simulink model "consigna_5_2"  (R2024b)
settings: Solver=ode45  StartTime=0.0  StopTime=600  FixedStep=1/39789  MaxStep=1e-1  RelTol=1e-5
InitFcn:
  | parametros
values from neighbouring files (symbols this model uses):
  A_corrientes = [0 1; -omega_n_corrientes^2 -2*omega_n_corrientes]    [parametros.m]
  A_inversor = [0 1; -omega_n_inversor^2 -2*omega_n_inversor]    [parametros.m]
  A_posicion = [0 1; -omega_n_posicion^2 -2*omega_n_posicion]    [parametros.m]
  A_temp = -1/20    (= -0.05)    [parametros.m]
  alpha_cu = 3.9 *10^-3    (= 0.0039)    [parametros.m]
  B_corrientes = [0; omega_n_corrientes^2]    [parametros.m]
  B_inversor = [0; omega_n_inversor^2]    [parametros.m]
  b_l = 0.1    [parametros.m]
  b_m = 1.5 * 10^-5    (= 1.5e-05)    [parametros.m]
  B_posicion = [0; omega_n_posicion^2]    [parametros.m]
  B_temp = 1/20    (= 0.05)    [parametros.m]
  ba = J_eq*n*omega_pos    (= 0.0395694444444)    [parametros.m]
  C_corrientes = [1 0]    [parametros.m]
  C_inversor = [1 0]    [parametros.m]
  C_posicion = [1 0]    [parametros.m]
  C_temp = 1    [parametros.m]
  C_ts = 0.818    [parametros.m]
  J_l = (m*l_cm^2 + J_cm) + (m_l * l_l^2)    (= 0.0833)    [parametros.m]
  J_m = 1.4 * 10^-5    (= 1.4e-05)    [parametros.m]
  K_e_int = 3200 ^3    (= 32768000000)    [parametros.m]
  K_e_omega = 3*3200^2    (= 30720000)    [parametros.m]
  K_e_theta = 9600    [parametros.m]
  k_l = m * g * l_cm + m_l * g * l_l    (= 2.4516625)    [parametros.m]
  Ksa = J_eq*n*(omega_pos^2)    (= 31.6555555556)    [parametros.m]
  Ksia = J_eq*(omega_pos^3)    (= 10129.7777778)    [parametros.m]
  L_d = 6.6 * 10^-3    (= 0.0066)    [parametros.m]
  L_ls = 0.8 * 10^-3    (= 0.0008)    [parametros.m]
  L_q = 5.8 * 10^-3    (= 0.0058)    [parametros.m]
  lambda_m = 0.016    [parametros.m]
  P_p = 3    [parametros.m]
  r = 120    [parametros.m]
  R_s_40 = 1.02    [parametros.m]
  R_ts_amb = 146.7    [parametros.m]
  T_sample = 1/f_sample    (= 4.53514739229e-05)    [parametros.m]
  Temp_s_ref = 20    [parametros.m]
  tm = X(1)    [parametros.m]
  tr = X(2)    [parametros.m]
  w1 = 2*pi*r/5    (= 150.796447372)    [parametros.m]
  x0_corrientes = [0;0]    [parametros.m]
  x0_inversor = [0;0]    [parametros.m]
  x0_posicion = [0; 0]    [parametros.m]
  x0_temp = 25    [parametros.m]
libraries: simulink x23, dspsigops x6
(part 1 of 5)
settings Model: SimulationMode=accelerator  Creator=Usuario  LastModifiedBy=gabri
settings DebuggingCC: AlgebraicLoopMsg=none

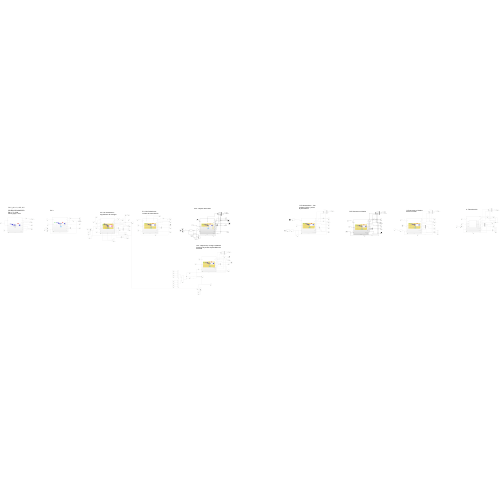
[thumbnail: Simulink's stored preview of the top-level diagram]
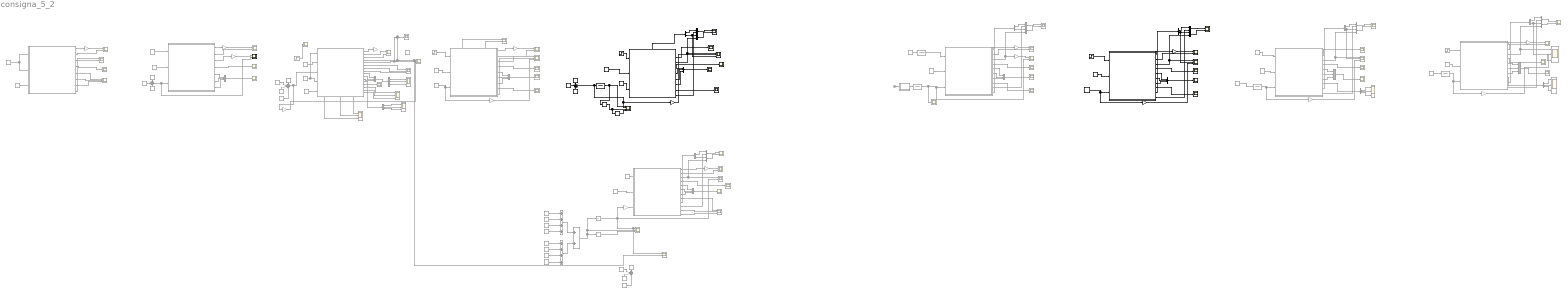
== system consigna_5_2 ==
  note: 5.2.1 i_ds* = 0, +0.5, -0.5
      |
      | PRUEBA SEGUIMIENTO TM* -> TL CON THETA_M(0) = PI/4
  note: 5.2.4 sin limitaciones - seguimiento de consigna
  note: 5.2.4 sin limitaciones - rechazo de perturbación
  note: 5.2.5 - Mejoras de consigna mediante formación de perfiles trapezoidales de velocidad
  note: 5.2.5 calentamiento - 10m consigna ciclica + pulsos de perturbación
  note: 5.2.5 Sensores no ideales
  note: 5.2.5 sensores no ideales inversor no ideal
  note: 6 - Discretización
  note: 5.2.3
  note: 5.2.5 - Mejora observador
  .5s : Step  Commented=on  Time=.5  After=5  SampleTime=0
  0-1 : simulink/Sources/Ramp  Commented=on  slope=2*pi/5  start=0  InitialOutput=0
  0-2 : simulink/Sources/Ramp  slope=2*pi/5  start=0  InitialOutput=0
  0-3 : simulink/Sources/Ramp  Commented=on  slope=2*pi/5  start=15  InitialOutput=0
  0-4 : simulink/Sources/Ramp  Commented=on  slope=2*pi/5  start=0  InitialOutput=0
  0-5 : simulink/Sources/Ramp  Commented=on  slope=2*pi/5  start=0  InitialOutput=0
  0-6 : simulink/Sources/Ramp  Commented=on  slope=2*pi/5  start=15  InitialOutput=0
  10-1 : simulink/Sources/Ramp  Commented=on  slope=-2*pi/5  start=10  InitialOutput=0
  10-15 : simulink/Sources/Ramp  Commented=on  slope=-2*pi/5  start=10  InitialOutput=0
  10-2 : simulink/Sources/Ramp  slope=-2*pi/5  start=10  InitialOutput=0
  10-3 : simulink/Sources/Ramp  Commented=on  slope=-2*pi/5  start=10  InitialOutput=0
  5-1 : simulink/Sources/Ramp  Commented=on  slope=-2*pi/5  start=5  InitialOutput=0
  5-10 : simulink/Sources/Ramp  Commented=on  slope=-2*pi/5  start=5  InitialOutput=0
  5-2 : simulink/Sources/Ramp  slope=-2*pi/5  start=5  InitialOutput=0
  5-3 : simulink/Sources/Ramp  Commented=on  slope=-2*pi/5  start=5  InitialOutput=0
  "5.2.1 " : Subsystem  Commented=on
  5.2.3 : Subsystem  Commented=on
  5.2.4 : Subsystem  Commented=on
      settings: PortSchema="{\"entries\":[{\"content\":{\"sides\":[{\"content\":{\"connectorIds\":[\"In1\",\"In2\",\"In3\",\"In4\",\"In5\"]},\"type\":\"ConnectorPlacement.EquallySpacedRectSide\",\"uuid\":\"f25aa34c-6f67-484c-a229-f52c6eeecdf1\"},{\"content\":{\"connectorIds\":[\"Out1\",\"Out2\",\"Out3\",\"Out4\",\"Out5\",\"Out6\",\"Out7\",\"Out8\",\"Out9\",\"Out10\",\"Out11\",\"Out12\",\"Out13\",\"Out14\",\"Out15\",\"Out16\"],\"side\":\"RIGHT\"},\"type\":\"ConnectorPlacement.EquallySpacedRectSide\",\"uuid\":\"6aed1817-4278-445a-93c2-caff5363bf6f\"},{\"content\":{\"side\":\"TOP\"},\"type\":\"ConnectorPlacement.EquallySpacedRectSide\",\"uuid\":\"7cbfa292-0843-4ea0-b7b1-1b35692a06de\"},{\"content\":{\"connectorIds\":[\"Out17\",\"Out18\",\"Out19\"],\"side\":\"BOTTOM\"},\"type\":\"ConnectorPlacement.EquallySpacedRectSide\",\"uuid\":\"b199e458-5f17-4edf-b279-750495dc0f0e\"}]},\"type\":\"ConnectorPlacement.EquallySpacedConnector\",\"uuid\":\"19aabd2c-ee83-4195-b5ac-13c3d5f141f0\"}],\"packageUris\":[\"http://schema.mathworks.com/mf0/Connector/R2020b\"],\"version\":\"1.0\"}"
  5.2.4.b : Subsystem  Commented=on
      settings: PortSchema="{\"entries\":[{\"content\":{\"sides\":[{\"content\":{\"connectorIds\":[\"In1\",\"In2\",\"In3\"]},\"type\":\"ConnectorPlacement.EquallySpacedRectSide\",\"uuid\":\"8b25de47-475f-4287-8ae4-53eaf326d459\"},{\"content\":{\"connectorIds\":[\"Out1\",\"Out2\",\"Out3\",\"Out4\",\"Out5\",\"Out6\",\"Out7\",\"Out8\",\"Out9\"],\"side\":\"RIGHT\"},\"type\":\"ConnectorPlacement.EquallySpacedRectSide\",\"uuid\":\"f06d5897-8e36-455d-9b67-4a95e7a5221c\"},{\"content\":{\"connectorIds\":[\"Out10\",\"Out11\"],\"side\":\"TOP\"},\"type\":\"ConnectorPlacement.EquallySpacedRectSide\",\"uuid\":\"fe71d55b-b6d0-46da-a788-438a4a7d80b0\"}]},\"type\":\"ConnectorPlacement.EquallySpacedConnector\",\"uuid\":\"95d0947e-b21b-4577-be3e-7cfd2e0895b9\"}],\"packageUris\":[\"http://schema.mathworks.com/mf0/Connector/R2020b\"],\"version\":\"1.0\"}"
  5.2.5 : Subsystem
      settings: PortSchema="{\"entries\":[{\"content\":{\"sides\":[{\"content\":{\"connectorIds\":[\"In1\",\"In2\",\"In3\"]},\"type\":\"ConnectorPlacement.EquallySpacedRectSide\",\"uuid\":\"8b25de47-475f-4287-8ae4-53eaf326d459\"},{\"content\":{\"connectorIds\":[\"Out1\",\"Out2\",\"Out3\",\"Out4\",\"Out5\",\"Out6\",\"Out7\",\"Out8\",\"Out9\"],\"side\":\"RIGHT\"},\"type\":\"ConnectorPlacement.EquallySpacedRectSide\",\"uuid\":\"f06d5897-8e36-455d-9b67-4a95e7a5221c\"},{\"content\":{\"connectorIds\":[\"Out10\"],\"side\":\"TOP\"},\"type\":\"ConnectorPlacement.EquallySpacedRectSide\",\"uuid\":\"fe71d55b-b6d0-46da-a788-438a4a7d80b0\"}]},\"type\":\"ConnectorPlacement.EquallySpacedConnector\",\"uuid\":\"95d0947e-b21b-4577-be3e-7cfd2e0895b9\"}],\"packageUris\":[\"http://schema.mathworks.com/mf0/Connector/R2020b\"],\"version\":\"1.0\"}"
  5.2.5' : Subsystem  Commented=on
  5.2.5.c : Subsystem  Commented=on
  5.2.5.d : Subsystem
  5.2.5.e : Subsystem  Commented=on
  Clock : Clock  Commented=on
  Constant{,1,6,10..11} (5 alike) : Constant  Commented=on  Value=20
  Constant12 : Constant  Commented=on  Value=40
  Constant13 : Constant  Value=20
  Constant14 : Constant  Commented=on  Value=40
  Constant{3..4,15,17..22} (9 alike) : Constant  Commented=on  Value=0
  Constant16 : Constant  Value=0
  Constant2 : Constant  Commented=on  Value=40
  Constant5 : Constant  Value=20
  Constant9 : Constant  Value=0
  Demux : Demux  Outputs=2
  Demux{6..8,10} (4 alike) : Demux  Commented=on  Outputs=3
  Demux{2..3,5,9} (4 alike) : Demux  Commented=on  Outputs=2
  Demux4 : Demux  Outputs=2
  Derivative : Derivative
  Derivative1 : Derivative
  Derivative2 : Derivative  Commented=on
  Error de observador : Scope  NumInputPorts=2
  Error de observador{2..3,5..6} (4 alike) : Scope  Commented=on  NumInputPorts=2
  Error de observador4 : Scope  NumInputPorts=2
  Gain{,4..6,8,14..15,20..21,36} (10 alike) : Gain  Commented=on  Gain=1/r
  Gain{1,28,30,32} (4 alike) : Gain  Commented=on  Gain=r
  Gain2 : Gain  Gain=r
  Gain3 : Gain  Gain=r
  Gain7 : Gain  Gain=1/r
  Integrator : Integrator  Commented=on
  MATLAB Function : MATLAB Function  Commented=on  TreatAsAtomicUnit=on
  Mux{,4,14,16} (4 alike) : Mux  Inputs=2
  Mux{1..2,9,12,18,21,41} (7 alike) : Mux  Commented=on  Inputs=3
  Mux{8,10..11,13,17,19..20,22} (8 alike) : Mux  Commented=on  Inputs=2
  Mux15 : Mux  Inputs=3
  Mux3 : Mux  Inputs=3
  Posición y velocidad : Scope  Commented=on  NumInputPorts=2
  Pulse Generator : DiscretePulseGenerator  Commented=on  PulseType=Time based  Amplitude=5  Period=1  PulseWidth=50
  Ramp : simulink/Sources/Ramp  Commented=on  slope=3*pi  start=5  InitialOutput=0
  Ramp1 : simulink/Sources/Ramp  Commented=on  slope=-w1  start=15  InitialOutput=0
  Ramp2 : simulink/Sources/Ramp  Commented=on  slope=w1  start=10+tr+tm  InitialOutput=0
  Ramp3 : simulink/Sources/Ramp  Commented=on  slope=w1  start=10+tr  InitialOutput=0
  Ramp4 : simulink/Sources/Ramp  Commented=on  slope=-w1  start=10  InitialOutput=0
  Ramp5 : simulink/Sources/Ramp  Commented=on  slope=w1  start=5  InitialOutput=0
  Ramp6 : simulink/Sources/Ramp  Commented=on  slope=-w1  start=tr+tm  InitialOutput=0
  Ramp7 : simulink/Sources/Ramp  Commented=on  slope=-w1  start=tr  InitialOutput=0
  Ramp8 : simulink/Sources/Ramp  Commented=on  slope=w1  start=0  InitialOutput=0
  Scope : Scope  Commented=on  NumInputPorts=2
  Scope1 : Scope  NumInputPorts=4
  Scope11 : Scope  Commented=on
  Scope4 : Scope  Commented=on  NumInputPorts=3
  Step : Step  Time=7.5  After=5  SampleTime=0
  Step1 : Step  Commented=on  Time=7.5  After=5  SampleTime=0
  Step3 : Step  Commented=on  Time=7.5  After=5  SampleTime=0
  Step4 : Step  Time=7.5  After=5  SampleTime=0
  Subsystem : Subsystem  Commented=on
  Sum : Sum  Commented=on  Inputs=+++
  Sum{1,3,8,11} (4 alike) : Sum  Commented=on  Inputs=++++
  Sum2 : Sum  Commented=on  Inputs=|-+
  Sum6 : Sum  Inputs=+++
  Sum9 : Sum  Commented=on
  Temperatura : Scope  Commented=on
  Tensiones Virtuales : Scope  Commented=on  NumInputPorts=3
  Tensiones reales : Scope  Commented=on  NumInputPorts=3
  Tensiones1 : Scope  Commented=on
  Tensiones2 : Scope
  Tensiones4 : Scope  Commented=on  NumInputPorts=3
  Tensiones5 : Scope  Commented=on
  Tensiones6 : Scope
  Tensiones7 : Scope  Commented=on  NumInputPorts=3
  Tensiones8 : Scope  Commented=on  NumInputPorts=3
  Torque carga vs motor : Scope  Commented=on  NumInputPorts=2
  Transfer Fcn2 : TransferFcn  Numerator=[10]  Denominator=[1 10]
  Transfer Fcn3 : TransferFcn  Commented=on  Numerator=[100]  Denominator=[1 100]
  Transfer Fcn4 : TransferFcn  Commented=on  Numerator=[10]  Denominator=[1 10]
  Transfer Fcn5 : TransferFcn  Commented=on  Numerator=[10]  Denominator=[1 10]
  Transfer Fcn8 : TransferFcn  Commented=on  Numerator=[20]  Denominator=[1 20]
  corrientes : Scope  Commented=on  NumInputPorts=3
  corrientes virtuales : Scope  Commented=on  NumInputPorts=3
  corrientes{2..3,6..7,9..10} (6 alike) : Scope  Commented=on
  corrientes4 : Scope
  corrientes8 : Scope
  corrrientes reales : Scope  Commented=on  NumInputPorts=3
  error de posicion : Scope  Commented=on
  posicion : Scope  Commented=on  NumInputPorts=3
  posicion del brazo : Scope  NumInputPorts=2
  posicion del brazo5 : Scope  Commented=on  NumInputPorts=2
  posicion del brazo6 : Scope  Commented=on  NumInputPorts=2
  posicion del brazo7 : Scope  NumInputPorts=3
  posicion del brazo8 : Scope  Commented=on  NumInputPorts=3
  posicion del brazo9 : Scope  Commented=on  NumInputPorts=3
  posicion2 : Scope  NumInputPorts=3
  posicion3 : Scope  Commented=on  NumInputPorts=3
  temp{,1..2,5..6,8..9} (7 alike) : Scope  Commented=on
  temp3 : Scope
  temp7 : Scope
  tld : Scope  Commented=on
  torque{,1..2,5..6,9} (6 alike) : Scope  Commented=on  NumInputPorts=2
  torque3 : Scope
  torque7 : Scope  NumInputPorts=2
  torque8 : Scope  Commented=on
  "velocidad " : Scope  Commented=on  NumInputPorts=2
  velocidad del brazo : Scope  Commented=on  NumInputPorts=3
  wires:
  5.2.3/7(fcs) -> Mux41/3
  5.2.3/5(fas) -> Mux41/1
  5.2.3/6(fbs) -> Mux41/2
  Mux41/1 -> corrientes2/1
  5.2.3/3("theta_m ") -> Gain/1
  Constant/1 -> 5.2.3/2(Tº_amb)
  5.2.3/4(T_s) -> temp/1
  "5.2.1 "/3("theta_m ") -> Posición y velocidad/1  "theta_m"
  Constant6/1 -> "5.2.1 "/3(Tº_amb)
  "5.2.1 "/7(fcs) -> corrientes/3  "i_cs"
  "5.2.1 "/6(fbs) -> corrientes/2  "i_bs"
  "5.2.1 "/2(T_m) -> Torque carga vs motor/2  "T_m"
  "5.2.1 "/5(fas) -> corrientes/1  "i_as"
  "5.2.1 "/4(T_s) -> Temperatura/1  "T_s"
  5.2.3/2(T_m) -> torque/2
  Sum/1 -> posicion del brazo/2, 5.2.3/3(q1*)  "q1*"
  0-5/1 -> Sum/2
  Gain/1 -> posicion del brazo/1  "q1"
  5-10/1 -> Sum/1
  10-15/1 -> Sum/3
  5-1/1 -> Sum1/1
  0-1/1 -> Sum1/2
  5.2.4/2(T_m) -> torque1/1  "Tm"
  5.2.4/4("theta_m ") -> Sum2/2, Scope/2, posicion/1  "theta_m"
  10-1/1 -> Sum1/3
  Mux1/1 -> Demux7/1
  5.2.4/13(T_s) -> temp1/1
  5.2.4/11(fcs) -> Mux1/3
  5.2.4/10(fbs) -> Mux1/2
  Constant1/1 -> 5.2.4/2(Tº_amb)
  5.2.4/9(fas) -> Mux1/1
  5.2.4/12(v_abcs) -> Demux6/1
  "5.2.1 "/8(omega_m) -> Posición y velocidad/2  "omega_m"
  5.2.4.b/5(fas) -> Mux2/1
  Step1/1 -> 5.2.4.b/1(T_per)  "T_per"
  Constant2/1 -> 5.2.4.b/2(Tº_amb)
  5.2.4.b/4(T_s) -> temp2/1
  5.2.4.b/2(T_m) -> torque2/2  "Tm"
  5.2.4.b/7(fcs) -> Mux2/3
  5.2.4.b/6(fbs) -> Mux2/2
  5.2.4.b/8(v_abcs) -> Tensiones1/1
  Mux2/1 -> corrientes3/1
  Constant3/1 -> Gain1/1, 5.2.4.b/3(q1*)  "q1*"
  Step3/1 -> tld/1
  Mux3/1 -> corrientes4/1  "i_abcs"
  5.2.5/7(fcs) -> Mux3/3  "ics"
  Sum6/1 -> Transfer Fcn2/1, Scope1/2, Gain2/1  "q1*"
  5.2.5/8(v_abcs) -> Tensiones2/1  "v_abcs"
  Constant5/1 -> 5.2.5/2(Tº_amb)
  5.2.5/5(fas) -> Mux3/1  "ias"
  5.2.5/6(fbs) -> Mux3/2  "ibs"
  5.2.5/2(T_m) -> torque3/1  "Tm"
  5.2.5/3("theta_m ") -> posicion2/1, Mux4/2  "theta_m"
  5.2.5/4(T_s) -> temp3/1  "T_s"
  Mux/1 -> Error de observador/1
  5.2.5/10(omega_theta_m_obs) -> Demux/1
  Demux/1 -> Mux/1  "omega_m_obs"
  5.2.5/9(omega_m) -> Mux/2  "omega_m"
  Demux/2 -> posicion2/3, Mux4/1  "theta_m_obs"
  Mux4/1 -> Error de observador/2
  5-2/1 -> Sum6/1
  0-2/1 -> Sum6/2
  10-2/1 -> Sum6/3
  Derivative/1 -> Derivative1/1, Scope1/3  "v"
  Derivative1/1 -> Scope1/4  "a"
  Constant9/1 -> 5.2.5/3(q1*)
  Transfer Fcn2/1 -> Scope1/1, Derivative/1  "q1* - suavizada"
  Transfer Fcn8/1 -> Scope11/1, posicion del brazo6/2, 5.2.5.c/3(q1*)  "q1*"
  Demux3/1 -> Mux13/1  "omega_m_obs"
  5.2.5.c/9(omega_m) -> Mux13/2  "omega_m"
  5.2.5.c/4(T_s) -> temp6/1  "T_s"
  5.2.5.c/10(omega_theta_obs) -> Demux3/1
  5.2.5.c/7(fcs) -> Mux12/3
  Mux12/1 -> corrientes7/1
  5.2.5.c/5(fas) -> Mux12/1
  5.2.5.c/8(v_abcs) -> Tensiones5/1
  Transfer Fcn3/1 -> 5.2.5.c/1(T_per)  "T_per"
  5.2.5.c/3("theta_m ") -> Mux11/2, Gain21/1  "theta_m"
  Demux3/2 -> Mux11/1  "theta_m_obs"
  Mux11/1 -> Error de observador3/2
  5.2.5.c/6(fbs) -> Mux12/2
  Mux13/1 -> Error de observador3/1
  5.2.5.c/2(T_m) -> torque6/2  "Tm"
  Gain21/1 -> posicion del brazo6/1  "q1"
  Constant11/1 -> 5.2.5.c/2(Tº_amb)
  Pulse Generator/1 -> Transfer Fcn3/1  "Tper"
  Demux4/2 -> posicion del brazo7/2, Mux14/1  "theta_m_obs"
  Constant13/1 -> 5.2.5.d/2(Tº_amb)
  5.2.5.d/3("theta_m ") -> Mux14/2, posicion del brazo7/1  "theta_m"
  5.2.5.d/2(T_m) -> torque7/2  "Tm"
  5.2.5.d/9(omega_theta_obs) -> Demux4/1
  5.2.5.d/4(T_s) -> temp7/1  "T_s"
  5.2.5.d/5(fas) -> Mux15/1  "i_as"
  5.2.5.d/6(fbs) -> Mux15/2  "i_bs"
  5.2.5.d/8(v_abcs) -> Tensiones6/1
  Step/1 -> 5.2.5.d/1(T_per)  "T_per"
  Mux14/1 -> Error de observador4/2
  Mux16/1 -> Error de observador4/1
  Mux15/1 -> corrientes8/1
  5.2.5.d/7(fcs) -> Mux15/3  "i_cs"
  5.2.5.d/10(omega_m) -> Mux16/2  "omega_m"
  5.2.4/6(omega_m_obs) -> velocidad del brazo/1  "omega_m_obs"
  5.2.4/7(omega_m) -> velocidad del brazo/2  "omega_m simulada"
  5.2.4/8(omega_m*) -> velocidad del brazo/3  "omega_m*"
  Demux6/1 -> Tensiones reales/1  "v_as"
  Demux6/2 -> Tensiones reales/2  "v_bs"
  Demux6/3 -> Tensiones reales/3  "v_cs"
  Demux7/1 -> corrrientes reales/1  "i_as"
  Demux7/2 -> corrrientes reales/2  "i_bs"
  Demux7/3 -> corrrientes reales/3  "i_cs"
  Clock/1 -> MATLAB Function/1(t)
  MATLAB Function/1(y) -> Transfer Fcn8/1
  Constant16/1 -> Gain3/1, 5.2.5.d/3(q1*)  "q1*"
  Gain3/1 -> posicion del brazo7/3  "theta_m*"
  Transfer Fcn4/1 -> Gain28/1, 5.2.5.e/3(q1*)  "q1*"
  Gain28/1 -> posicion del brazo8/3  "theta_m*"
  Mux19/1 -> Error de observador5/1
  5.2.5.e/8(v_abcs) -> Demux8/1
  5.2.5.e/5(fas) -> Mux18/1  "i_as"
  5.2.5.e/6(fbs) -> Mux18/2  "i_bs"
  Demux5/2 -> posicion del brazo8/2, Mux17/1  "theta_m_obs"
  Demux5/1 -> Mux19/1  "omega_m_obs"
  Mux17/1 -> Error de observador5/2
  5.2.5.e/10(omega_m) -> Mux19/2  "omega_m"
  Mux18/1 -> corrientes9/1
  5.2.5.e/3("theta_m ") -> Mux17/2, posicion del brazo8/1  "theta_m"
  5.2.5.e/7(fcs) -> Mux18/3  "i_cs"
  Constant15/1 -> 5.2.5.e/1(T_per)  "T_per"
  Constant12/1 -> 5.2.5.e/2(Tº_amb)
  5.2.5.e/2(T_m) -> torque8/1  "Tm"
  5.2.5.e/9(omega_theta_obs) -> Demux5/1
  5.2.5.e/4(T_s) -> temp8/1  "T_s"
  Ramp/1 -> Transfer Fcn4/1  "q1*"
  Demux8/1 -> Tensiones7/1  "v_as"
  Demux8/2 -> Tensiones7/2  "v_bs"
  Demux8/3 -> Tensiones7/3  "v_cs"
  Demux9/1 -> Mux22/1  "omega_m_obs"
  Mux20/1 -> Error de observador6/2
  Mux22/1 -> Error de observador6/1
  Mux21/1 -> corrientes10/1
  Demux9/2 -> posicion del brazo9/3, Mux20/1  "theta_m_obs"
  Gain32/1 -> posicion del brazo9/2  "theta_m*"
  Demux10/2 -> Tensiones8/2  "v_bs"
  Demux10/1 -> Tensiones8/1  "v_as"
  Constant20/1 -> Transfer Fcn5/1  "q1*"
  Demux10/3 -> Tensiones8/3  "v_cs"
  Transfer Fcn5/1 -> Subsystem/3(q1*), Gain32/1
  5.2.5'/4(T_s) -> temp5/1
  5.2.5'/9(omega_theta_obs) -> Demux2/1
  5.2.5'/2(T_m) -> torque5/2  "Tm"
  Mux9/1 -> corrientes6/1
  5.2.5'/7(fcs) -> Mux9/3  "ics"
  5.2.5'/10(omega_m) -> Mux8/2  "omega_m"
  5.2.5'/3("theta_m ") -> posicion del brazo5/1, Mux10/2  "theta_m"
  Constant18/1 -> 5.2.5'/1(T_per)
  Demux2/2 -> Mux10/1  "theta_m_obs"
  Mux10/1 -> Error de observador2/2
  Demux2/1 -> Mux8/1  "omega_m_obs"
  5.2.5'/6(fbs) -> Mux9/2  "ibs"
  5.2.5'/8(v_as) -> Tensiones4/1  "vas"
  Constant10/1 -> 5.2.5'/2(Tº_amb)
  5.2.5'/5(fas) -> Mux9/1  "ias"
  Mux8/1 -> Error de observador2/1
  Ramp1/1 -> Sum8/1
  Ramp4/1 -> Sum8/4
  Ramp3/1 -> Sum8/3
  Ramp2/1 -> Sum8/2
  Ramp8/1 -> Sum11/4
  Ramp7/1 -> Sum11/3
  Ramp6/1 -> Sum11/2
  Ramp5/1 -> Sum11/1
  Sum8/1 -> Sum9/1
  Sum11/1 -> Sum9/2
  Sum9/1 -> Derivative2/1, Integrator/1, Scope4/2  "vel"
  Integrator/1 -> posicion del brazo5/2, Gain36/1, Scope/1, Scope4/1  "Consigna de Posicion"
  Derivative2/1 -> Scope4/3  "acel"
  Constant17/1 -> 5.2.3/1(T_per)
  "5.2.1 "/1(T_l) -> Gain4/1
  Constant19/1 -> "5.2.1 "/1(Tm*), "5.2.1 "/2(T_per)
  5.2.4.b/1(T_l) -> Gain15/1
  5.2.4.b/9(theta_m_obs) -> posicion3/2  "theta_m_obs"
  5.2.4.b/3("theta_m ") -> posicion3/1  "theta_m"
  Gain1/1 -> posicion3/3  "theta_m*"
  Gain2/1 -> posicion2/2  "theta_m*"
  5.2.5'/1(T_l) -> Gain20/1
  Gain4/1 -> Torque carga vs motor/1  "T_l"
  5.2.3/1(T_l) -> Gain5/1
  Gain5/1 -> torque/1
  5.2.4/1(T_l) -> Gain14/1
  Gain15/1 -> torque2/1
  5.2.4.b/10(omega_m_simulada) -> "velocidad "/1
  5.2.4.b/11(omega_m_obs) -> "velocidad "/2
  Gain20/1 -> torque5/1  "q1"
  Gain36/1 -> 5.2.5'/3(q1*)
  5.2.5.c/1(T_l) -> Gain6/1
  Gain6/1 -> torque6/1  "q1"
  Demux4/1 -> Mux16/1
  5.2.5.d/1(T_l) -> Gain7/1
  Gain7/1 -> torque7/1  "theta_m*"
  Gain8/1 -> torque9/1
  Subsystem/3(theta_m) -> Mux20/2, posicion del brazo9/1  "theta_m muestreada"
  .5s/1 -> Subsystem/1(T_per)  "T_per"
  Constant14/1 -> Subsystem/2(Tº_amb)
  Subsystem/1(omega_m) -> Gain8/1
  Subsystem/2(Tm) -> torque9/2
  Subsystem/4(T_s) -> temp9/1  "T_s"
  Subsystem/5(i_as) -> Mux21/1
  Subsystem/6(i_bs) -> Mux21/2
  Subsystem/7(i_cs) -> Mux21/3
  Subsystem/8(v_abcs) -> Demux10/1
  Subsystem/9(omega_theta_obs) -> Demux9/1
  Subsystem/10(omega_m1) -> Mux22/2
  0-3/1 -> Sum1/4
  5.2.4/3(Tm*) -> torque1/2
  5.2.4/14(v_qs*') -> Tensiones Virtuales/1
  5.2.4/15(v_ds*') -> Tensiones Virtuales/2
  5.2.4/16(v_0s*') -> Tensiones Virtuales/3
  Constant21/1 -> 5.2.4/1(T_per), 5.2.4/4(I_ds*)
  Constant22/1 -> 5.2.4/5(I_0s*)
  5.2.4/19(iqs) -> corrientes virtuales/1
  5.2.4/18(ids) -> corrientes virtuales/2
  5.2.4/17(i0s) -> corrientes virtuales/3
  5.2.4/5(theta_m_obs) -> Sum2/1, posicion/2  "theta_m_obs"
  Sum2/1 -> error de posicion/1
  Sum1/1 -> Gain30/1, 5.2.4/3(q1*)  "q1*"
  Gain30/1 -> posicion/3  "theta_m*"
  10-3/1 -> Sum3/3
  0-6/1 -> Sum3/4
  0-4/1 -> Sum3/2
  5-3/1 -> Sum3/1
  5.2.5'/11(v_bs) -> Tensiones4/2  "vbs"
  5.2.5'/12(v_cs) -> Tensiones4/3  "vcs"
  Step4/1 -> 5.2.5/1(T_per)  "Tper"

== system consigna_5_2/5.2.1  ==
  Tm* : Inport
  T_per : Inport  Port=2
  Tº_amb : Inport  Port=3
  Calculo rs : Subsystem
  Constant5 : Constant  Value=0
  Demux : Demux  Outputs=3
  Desacoplamientos físicos : Subsystem
  Desacoplamientos físicos de torque : Subsystem
  Gain5 : Gain  Gain=P_p
  Modulador de corriente : Subsystem
  Modulador de tensión : Subsystem
  Modulador de torque : Subsystem
  Sensores : Subsystem
  Subsistema físico no lineal : Subsystem
      settings: PortSchema="{\"entries\":[{\"content\":{\"sides\":[{\"content\":{\"connectorIds\":[\"In1\",\"In2\",\"In3\",\"In4\",\"In5\"]},\"type\":\"ConnectorPlacement.EquallySpacedRectSide\",\"uuid\":\"67117692-d9ee-40bf-88b2-d8f6a60dc3b5\"},{\"content\":{\"connectorIds\":[\"Out1\",\"Out2\",\"Out3\"],\"side\":\"RIGHT\"},\"type\":\"ConnectorPlacement.EquallySpacedRectSide\",\"uuid\":\"ca2dbe86-e86f-47c7-8eac-1e82e6a5dbc0\"},{\"content\":{\"connectorIds\":[\"Out4\",\"Out5\",\"Out6\"],\"side\":\"TOP\"},\"type\":\"ConnectorPlacement.EquallySpacedRectSide\",\"uuid\":\"fbd4a5c3-5162-48dd-8002-932f8e6631f6\"}]},\"type\":\"ConnectorPlacement.EquallySpacedConnector\",\"uuid\":\"e55c07f0-88b9-4508-920f-2bf50421126b\"}],\"packageUris\":[\"http://schema.mathworks.com/mf0/Connector/R2020b\"],\"version\":\"1.0\"}"
  TD_PARK : MATLAB Function  TreatAsAtomicUnit=on
  TI_PARK1 : MATLAB Function  TreatAsAtomicUnit=on
  T_l : Outport
  T_m : Outport  Port=2
  "theta_m " : Outport  Port=3
  T_s : Outport  Port=4
  fas : Outport  Port=5
  fbs : Outport  Port=6
  fcs : Outport  Port=7
  omega_m : Outport  Port=8
  wires:
  Modulador de tensión/1(v_as) -> Subsistema físico no lineal/2(v_as)
  TD_PARK/3(f0s) -> Desacoplamientos físicos/6(i_0s), Modulador de corriente/6(i_0s)  "i_0s"
  TI_PARK1/1(fas) -> Modulador de tensión/1(v_as*)
  Sensores/2(T_s_medida) -> T_s/1, Calculo rs/1(Ts)
  Modulador de tensión/2(v_bs) -> Subsistema físico no lineal/3(v_bs)
  TD_PARK/1(fqs) -> Modulador de corriente/4(i_qs), Desacoplamientos físicos/4(i_qs)  "i_qs^r"
  Sensores/1(theta_m_medida) -> "theta_m "/1, Desacoplamientos físicos de torque/2(theta_m), Gain5/1
  TI_PARK1/2(fbs) -> Modulador de tensión/2(v_bs*)
  TD_PARK/2(fds) -> Modulador de torque/2(ids), Desacoplamientos físicos/5(i_ds), Modulador de corriente/5(i_ds)  "i_ds^r"
  Desacoplamientos físicos/3(v_0s*') -> TI_PARK1/3(f0s)
  Modulador de tensión/3(v_cs) -> Subsistema físico no lineal/4(v_cs)
  Subsistema físico no lineal/1(theta_m) -> Sensores/1(theta_m)
  Subsistema físico no lineal/2(T_s) -> Sensores/2(T_s)
  Sensores/5(i_cs_medida) -> fcs/1, TD_PARK/3(fcs)
  Demux/1 -> Sensores/3(i_as)
  Modulador de torque/1(iq*) -> Modulador de corriente/1(I_qs*)
  Gain5/1 -> TD_PARK/4(theta_r), TI_PARK1/4(theta_r)
  Sensores/4(i_bs_medida) -> fbs/1, TD_PARK/2(fbs)
  Modulador de corriente/1(v_qs*) -> Desacoplamientos físicos/1(v_qs*)
  Constant5/1 -> Modulador de corriente/3(I_0s*), Modulador de corriente/2(I_ds*)
  T_per/1 -> Subsistema físico no lineal/1(T_per)
  Demux/2 -> Sensores/4(i_bs)
  Modulador de corriente/3(v_0s*) -> Desacoplamientos físicos/3(v_0s*)
  Demux/3 -> Sensores/5(i_cs)
  Desacoplamientos físicos/1(v_qs*') -> TI_PARK1/1(fqs)
  Sensores/3(i_as_medida) -> TD_PARK/1(fas), fas/1
  TI_PARK1/3(fcs) -> Modulador de tensión/3(v_cs*)
  Tº_amb/1 -> Subsistema físico no lineal/5(Tº_amb), Calculo rs/2(Tamb)
  Desacoplamientos físicos/2(v_ds*') -> TI_PARK1/2(fds)
  Modulador de corriente/2(v_ds*) -> Desacoplamientos físicos/2(v_ds*)
  Calculo rs/1(r_s) -> Desacoplamientos físicos/8(r_s)
  Desacoplamientos físicos de torque/1(Tm*') -> Modulador de torque/1(Tm*)
  Tm*/1 -> Desacoplamientos físicos de torque/1(Tm*)
  Subsistema físico no lineal/3(i_abcs) -> Demux/1
  Subsistema físico no lineal/4(omega_m) -> Modulador de torque/3(omega_m), Desacoplamientos físicos/7(omega_m), omega_m/1
  Subsistema físico no lineal/5(T_m) -> T_m/1
  Subsistema físico no lineal/6(T_l) -> T_l/1

== system consigna_5_2/5.2.3 ==
  T_per : Inport
  Tº_amb : Inport  Port=2
  q1* : Inport  Port=3
  Calculo rs : Subsystem
  Constant5 : Constant  Value=0
  Controlador PID : Subsystem
  Demux : Demux  Outputs=3
  Desacoplamientos físicos : Subsystem
  Desacoplamientos físicos de torque : Subsystem
  Gain5 : Gain  Gain=P_p
  Modulador de corriente : Subsystem
  Modulador de tensión : Subsystem
  Modulador de torque : Subsystem
  Observador de estado reducido : Subsystem
  Sensores : Subsystem
  Setpoint : Subsystem
  Subsistema físico no lineal : Subsystem
      settings: PortSchema="{\"entries\":[{\"content\":{\"sides\":[{\"content\":{\"connectorIds\":[\"In1\",\"In2\",\"In3\",\"In4\",\"In5\"]},\"type\":\"ConnectorPlacement.EquallySpacedRectSide\",\"uuid\":\"67117692-d9ee-40bf-88b2-d8f6a60dc3b5\"},{\"content\":{\"connectorIds\":[\"Out1\",\"Out2\",\"Out3\"],\"side\":\"RIGHT\"},\"type\":\"ConnectorPlacement.EquallySpacedRectSide\",\"uuid\":\"ca2dbe86-e86f-47c7-8eac-1e82e6a5dbc0\"},{\"content\":{\"connectorIds\":[\"Out4\",\"Out5\",\"Out6\"],\"side\":\"TOP\"},\"type\":\"ConnectorPlacement.EquallySpacedRectSide\",\"uuid\":\"fbd4a5c3-5162-48dd-8002-932f8e6631f6\"}]},\"type\":\"ConnectorPlacement.EquallySpacedConnector\",\"uuid\":\"e55c07f0-88b9-4508-920f-2bf50421126b\"}],\"packageUris\":[\"http://schema.mathworks.com/mf0/Connector/R2020b\"],\"version\":\"1.0\"}"
  TD_PARK : MATLAB Function  TreatAsAtomicUnit=on
  TI_PARK1 : MATLAB Function  TreatAsAtomicUnit=on
  T_l : Outport
  T_m : Outport  Port=2
  "theta_m " : Outport  Port=3
  T_s : Outport  Port=4
  fas : Outport  Port=5
  fbs : Outport  Port=6
  fcs : Outport  Port=7
  wires:
  Modulador de tensión/1(v_as) -> Subsistema físico no lineal/2(v_as)
  TD_PARK/3(f0s) -> Modulador de corriente/6(i_0s), Desacoplamientos físicos/6(i_0s)  "i_0s"
  TI_PARK1/1(fas) -> Modulador de tensión/1(v_as*)
  Modulador de tensión/2(v_bs) -> Subsistema físico no lineal/3(v_bs)
  TD_PARK/1(fqs) -> Modulador de corriente/4(i_qs), Desacoplamientos físicos/4(i_qs)  "i_qs^r"
  Gain5/1 -> TD_PARK/4(theta_r), TI_PARK1/4(theta_r)
  TI_PARK1/2(fbs) -> Modulador de tensión/2(v_bs*)
  TD_PARK/2(fds) -> Modulador de torque/2(ids), Modulador de corriente/5(i_ds), Desacoplamientos físicos/5(i_ds)  "i_ds^r"
  Desacoplamientos físicos/3(v_0s*') -> TI_PARK1/3(f0s)
  Modulador de tensión/3(v_cs) -> Subsistema físico no lineal/4(v_cs)
  Subsistema físico no lineal/1(theta_m) -> Sensores/1(theta_m)
  Subsistema físico no lineal/2(T_s) -> Sensores/2(T_s)
  Sensores/5(i_cs_medida) -> fcs/1, TD_PARK/3(fcs)
  Demux/1 -> Sensores/3(i_as)
  Modulador de torque/1(iq*) -> Modulador de corriente/1(I_qs*)
  Sensores/4(i_bs_medida) -> fbs/1, TD_PARK/2(fbs)
  Subsistema físico no lineal/5(T_m) -> T_m/1
  Modulador de corriente/1(v_qs*) -> Desacoplamientos físicos/1(v_qs*)
  Constant5/1 -> Modulador de corriente/3(I_0s*), Modulador de corriente/2(I_ds*)
  T_per/1 -> Subsistema físico no lineal/1(T_per)
  Demux/2 -> Sensores/4(i_bs)
  Modulador de corriente/3(v_0s*) -> Desacoplamientos físicos/3(v_0s*)
  Demux/3 -> Sensores/5(i_cs)
  Sensores/1(theta_m_medida) -> "theta_m "/1, Observador de estado reducido/2(theta_m), Gain5/1
  Desacoplamientos físicos/1(v_qs*') -> TI_PARK1/1(fqs)
  Sensores/3(i_as_medida) -> TD_PARK/1(fas), fas/1
  TI_PARK1/3(fcs) -> Modulador de tensión/3(v_cs*)
  Desacoplamientos físicos/2(v_ds*') -> TI_PARK1/2(fds)
  Modulador de corriente/2(v_ds*) -> Desacoplamientos físicos/2(v_ds*)
  Setpoint/2(omega_m*) -> Controlador PID/1(omega_m*)
  q1*/1 -> Setpoint/1(q1*)
  Controlador PID/1(Tm*) -> Observador de estado reducido/1(T_m*), Desacoplamientos físicos de torque/1(Tm*)
  Observador de estado reducido/1(omega_m_obs) -> Modulador de torque/3(omega_m), Controlador PID/2(omega_m), Desacoplamientos físicos/7(omega_m)
  Tº_amb/1 -> Subsistema físico no lineal/5(Tº_amb)
  Sensores/2(T_s_medida) -> Calculo rs/1(Ts), T_s/1
  Calculo rs/1(r_s) -> Desacoplamientos físicos/8(r_s)
  Desacoplamientos físicos de torque/1(Tm*') -> Modulador de torque/1(Tm*)
  Observador de estado reducido/2(theta_m_obs) -> Desacoplamientos físicos de torque/2(theta_m)
  Subsistema físico no lineal/3(i_abcs) -> Demux/1
  Subsistema físico no lineal/6(T_l) -> T_l/1

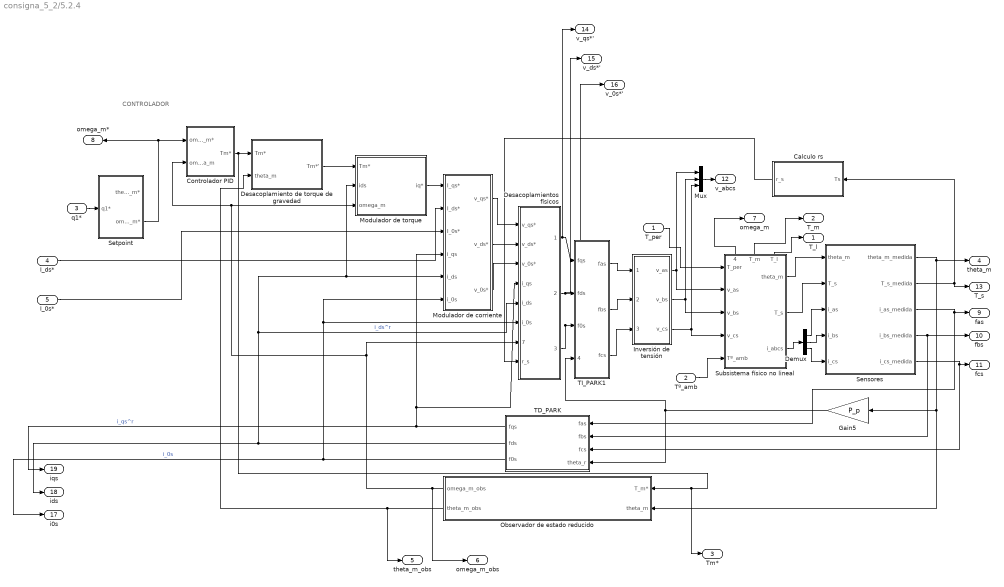
== system consigna_5_2/5.2.4 ==
  note: CONTROLADOR
  T_per : Inport
  Tº_amb : Inport  Port=2
  q1* : Inport  Port=3
  I_ds* : Inport  Port=4
  I_0s* : Inport  Port=5
  Calculo rs : Subsystem
  Controlador PID : Subsystem
  Demux : Demux  Outputs=3
  Desacoplamiento de torque de gravedad : Subsystem
  Desacoplamientos físicos : Subsystem
  Gain5 : Gain  Gain=P_p
  Inversión de tensión : Subsystem
  Modulador de corriente : Subsystem
  Modulador de torque : Subsystem
  Mux : Mux  Inputs=3
  Observador de estado reducido : Subsystem
  Sensores : Subsystem
  Setpoint : Subsystem
  Subsistema físico no lineal : Subsystem
      settings: PortSchema="{\"entries\":[{\"content\":{\"sides\":[{\"content\":{\"connectorIds\":[\"In1\",\"In2\",\"In3\",\"In4\",\"In5\"]},\"type\":\"ConnectorPlacement.EquallySpacedRectSide\",\"uuid\":\"67117692-d9ee-40bf-88b2-d8f6a60dc3b5\"},{\"content\":{\"connectorIds\":[\"Out1\",\"Out2\",\"Out3\"],\"side\":\"RIGHT\"},\"type\":\"ConnectorPlacement.EquallySpacedRectSide\",\"uuid\":\"ca2dbe86-e86f-47c7-8eac-1e82e6a5dbc0\"},{\"content\":{\"connectorIds\":[\"Out4\",\"Out5\",\"Out6\"],\"side\":\"TOP\"},\"type\":\"ConnectorPlacement.EquallySpacedRectSide\",\"uuid\":\"fbd4a5c3-5162-48dd-8002-932f8e6631f6\"}]},\"type\":\"ConnectorPlacement.EquallySpacedConnector\",\"uuid\":\"e55c07f0-88b9-4508-920f-2bf50421126b\"}],\"packageUris\":[\"http://schema.mathworks.com/mf0/Connector/R2020b\"],\"version\":\"1.0\"}"
  TD_PARK : MATLAB Function  TreatAsAtomicUnit=on
  TI_PARK1 : MATLAB Function  TreatAsAtomicUnit=on
  T_l : Outport
  T_m : Outport  Port=2
  Tm* : Outport  Port=3
  "theta_m " : Outport  Port=4
  theta_m_obs : Outport  Port=5
  omega_m_obs : Outport  Port=6
  omega_m : Outport  Port=7
  omega_m* : Outport  Port=8
  fas : Outport  Port=9
  fbs : Outport  Port=10
  fcs : Outport  Port=11
  v_abcs : Outport  Port=12
  T_s : Outport  Port=13
  v_qs*' : Outport  Port=14
  v_ds*' : Outport  Port=15
  v_0s*' : Outport  Port=16
  i0s : Outport  Port=17
  ids : Outport  Port=18
  iqs : Outport  Port=19
  wires:
  Inversión de tensión/1(v_as) -> Subsistema físico no lineal/2(v_as), Mux/1
  TD_PARK/3(f0s) -> i0s/1, Modulador de corriente/6(i_0s), Desacoplamientos físicos/6(i_0s)  "i_0s"
  TI_PARK1/1(fas) -> Inversión de tensión/1(v_as*)
  Inversión de tensión/2(v_bs) -> Subsistema físico no lineal/3(v_bs), Mux/2
  TD_PARK/1(fqs) -> iqs/1, Modulador de corriente/4(i_qs), Desacoplamientos físicos/4(i_qs)  "i_qs^r"
  Gain5/1 -> TI_PARK1/4(theta_r), TD_PARK/4(theta_r)
  TI_PARK1/2(fbs) -> Inversión de tensión/2(v_bs*)
  TD_PARK/2(fds) -> ids/1, Modulador de corriente/5(i_ds), Modulador de torque/2(ids), Desacoplamientos físicos/5(i_ds)  "i_ds^r"
  Desacoplamientos físicos/3(v_0s*') -> v_0s*'/1, TI_PARK1/3(f0s)
  Inversión de tensión/3(v_cs) -> Mux/3, Subsistema físico no lineal/4(v_cs)
  Subsistema físico no lineal/1(theta_m) -> Sensores/1(theta_m)
  Subsistema físico no lineal/2(T_s) -> Sensores/2(T_s)
  Sensores/5(i_cs_medida) -> TD_PARK/3(fcs), fcs/1
  Demux/1 -> Sensores/3(i_as)
  Modulador de torque/1(iq*) -> Modulador de corriente/1(I_qs*)
  Sensores/4(i_bs_medida) -> TD_PARK/2(fbs), fbs/1
  Subsistema físico no lineal/5(T_m) -> T_m/1
  Modulador de corriente/1(v_qs*) -> Desacoplamientos físicos/1(v_qs*)
  T_per/1 -> Subsistema físico no lineal/1(T_per)
  Demux/2 -> Sensores/4(i_bs)
  Modulador de corriente/3(v_0s*) -> Desacoplamientos físicos/3(v_0s*)
  Demux/3 -> Sensores/5(i_cs)
  Sensores/1(theta_m_medida) -> "theta_m "/1, Gain5/1, Observador de estado reducido/2(theta_m)
  Desacoplamientos físicos/1(v_qs*') -> v_qs*'/1, TI_PARK1/1(fqs)
  Sensores/3(i_as_medida) -> TD_PARK/1(fas), fas/1
  TI_PARK1/3(fcs) -> Inversión de tensión/3(v_cs*)
  Desacoplamientos físicos/2(v_ds*') -> v_ds*'/1, TI_PARK1/2(fds)
  Modulador de corriente/2(v_ds*) -> Desacoplamientos físicos/2(v_ds*)
  Setpoint/2(omega_m*) -> omega_m*/1, Controlador PID/1(omega_m*)
  q1*/1 -> Setpoint/1(q1*)
  Controlador PID/1(Tm*) -> Desacoplamiento de torque de gravedad/1(Tm*), Tm*/1, Observador de estado reducido/1(T_m*)
  Observador de estado reducido/1(omega_m_obs) -> omega_m_obs/1, Modulador de torque/3(omega_m), Controlador PID/2(omega_m), Desacoplamientos físicos/7(omega_m)
  Tº_amb/1 -> Subsistema físico no lineal/5(Tº_amb)
  Sensores/2(T_s_medida) -> T_s/1, Calculo rs/1(Ts)
  Calculo rs/1(r_s) -> Desacoplamientos físicos/8(r_s)
  Desacoplamiento de torque de gravedad/1(Tm*') -> Modulador de torque/1(Tm*)
  Observador de estado reducido/2(theta_m_obs) -> theta_m_obs/1, Desacoplamiento de torque de gravedad/2(theta_m)
  Mux/1 -> v_abcs/1
  Subsistema físico no lineal/4(omega_m) -> omega_m/1
  Subsistema físico no lineal/3(i_abcs) -> Demux/1
  Subsistema físico no lineal/6(T_l) -> T_l/1
  I_ds*/1 -> Modulador de corriente/2(I_ds*)
  I_0s*/1 -> Modulador de corriente/3(I_0s*)

== system consigna_5_2/5.2.4.b ==
  note: CONTROLADOR
  T_per : Inport
  Tº_amb : Inport  Port=2
  q1* : Inport  Port=3
  Calculo rs : Subsystem
  Constant5 : Constant  Value=0
  Controlador PID : Subsystem
  Demux : Demux  Outputs=3
  Desacoplamiento de torque de gravedad : Subsystem
  Desacoplamientos físicos : Subsystem
  Gain5 : Gain  Gain=P_p
  Inversión de tensión : Subsystem
  Modulador de corriente : Subsystem
  Modulador de torque : Subsystem
  Mux : Mux  Inputs=3
  Observador de estado reducido : Subsystem
  Sensores : Subsystem
  Setpoint : Subsystem
  Subsistema físico no lineal : Subsystem
      settings: PortSchema="{\"entries\":[{\"content\":{\"sides\":[{\"content\":{\"connectorIds\":[\"In1\",\"In2\",\"In3\",\"In4\",\"In5\"]},\"type\":\"ConnectorPlacement.EquallySpacedRectSide\",\"uuid\":\"67117692-d9ee-40bf-88b2-d8f6a60dc3b5\"},{\"content\":{\"connectorIds\":[\"Out1\",\"Out2\",\"Out3\"],\"side\":\"RIGHT\"},\"type\":\"ConnectorPlacement.EquallySpacedRectSide\",\"uuid\":\"ca2dbe86-e86f-47c7-8eac-1e82e6a5dbc0\"},{\"content\":{\"connectorIds\":[\"Out4\",\"Out5\",\"Out6\"],\"side\":\"TOP\"},\"type\":\"ConnectorPlacement.EquallySpacedRectSide\",\"uuid\":\"fbd4a5c3-5162-48dd-8002-932f8e6631f6\"}]},\"type\":\"ConnectorPlacement.EquallySpacedConnector\",\"uuid\":\"e55c07f0-88b9-4508-920f-2bf50421126b\"}],\"packageUris\":[\"http://schema.mathworks.com/mf0/Connector/R2020b\"],\"version\":\"1.0\"}"
  TD_PARK : MATLAB Function  TreatAsAtomicUnit=on
  TI_PARK1 : MATLAB Function  TreatAsAtomicUnit=on
  T_l : Outport
  T_m : Outport  Port=2
  "theta_m " : Outport  Port=3
  T_s : Outport  Port=4
  fas : Outport  Port=5
  fbs : Outport  Port=6
  fcs : Outport  Port=7
  v_abcs : Outport  Port=8
  theta_m_obs : Outport  Port=9
  omega_m_simulada : Outport  Port=10
  omega_m_obs : Outport  Port=11
  wires:
  Inversión de tensión/1(v_as) -> Subsistema físico no lineal/2(v_as), Mux/1
  TD_PARK/3(f0s) -> Modulador de corriente/6(i_0s), Desacoplamientos físicos/6(i_0s)  "i_0s"
  TI_PARK1/1(fas) -> Inversión de tensión/1(v_as*)
  Inversión de tensión/2(v_bs) -> Subsistema físico no lineal/3(v_bs), Mux/2
  TD_PARK/1(fqs) -> Modulador de corriente/4(i_qs), Desacoplamientos físicos/4(i_qs)  "i_qs^r"
  Gain5/1 -> TD_PARK/4(theta_r), TI_PARK1/4(theta_r)
  TI_PARK1/2(fbs) -> Inversión de tensión/2(v_bs*)
  TD_PARK/2(fds) -> Modulador de torque/2(ids), Modulador de corriente/5(i_ds), Desacoplamientos físicos/5(i_ds)  "i_ds^r"
  Desacoplamientos físicos/3(v_0s*') -> TI_PARK1/3(f0s)
  Inversión de tensión/3(v_cs) -> Subsistema físico no lineal/4(v_cs), Mux/3
  Subsistema físico no lineal/1(theta_m) -> Sensores/1(theta_m)
  Subsistema físico no lineal/2(T_s) -> Sensores/2(T_s)
  Sensores/5(i_cs_medida) -> fcs/1, TD_PARK/3(fcs)
  Demux/1 -> Sensores/3(i_as)
  Modulador de torque/1(iq*) -> Modulador de corriente/1(I_qs*)
  Sensores/4(i_bs_medida) -> fbs/1, TD_PARK/2(fbs)
  Subsistema físico no lineal/4(T_m) -> T_m/1
  Modulador de corriente/1(v_qs*) -> Desacoplamientos físicos/1(v_qs*)
  Constant5/1 -> Modulador de corriente/3(I_0s*), Modulador de corriente/2(I_ds*)
  T_per/1 -> Subsistema físico no lineal/1(T_per)
  Demux/2 -> Sensores/4(i_bs)
  Modulador de corriente/3(v_0s*) -> Desacoplamientos físicos/3(v_0s*)
  Demux/3 -> Sensores/5(i_cs)
  Sensores/1(theta_m_medida) -> "theta_m "/1, Observador de estado reducido/2(theta_m), Gain5/1
  Desacoplamientos físicos/1(v_qs*') -> TI_PARK1/1(fqs)
  Sensores/3(i_as_medida) -> TD_PARK/1(fas), fas/1
  TI_PARK1/3(fcs) -> Inversión de tensión/3(v_cs*)
  Desacoplamientos físicos/2(v_ds*') -> TI_PARK1/2(fds)
  Modulador de corriente/2(v_ds*) -> Desacoplamientos físicos/2(v_ds*)
  Setpoint/2(omega_m*) -> Controlador PID/1(omega_m*)
  q1*/1 -> Setpoint/1(q1*)
  Controlador PID/1(Tm*) -> Observador de estado reducido/1(T_m*), Desacoplamiento de torque de gravedad/1(Tm*)
  Observador de estado reducido/1(omega_m_obs) -> omega_m_obs/1, Modulador de torque/3(omega_m), Controlador PID/2(omega_m), Desacoplamientos físicos/7(omega_m)
  Tº_amb/1 -> Subsistema físico no lineal/5(Tº_amb)
  Sensores/2(T_s_medida) -> Calculo rs/1(Ts), T_s/1
  Calculo rs/1(r_s) -> Desacoplamientos físicos/8(r_s)
  Desacoplamiento de torque de gravedad/1(Tm*') -> Modulador de torque/1(Tm*)
  Observador de estado reducido/2(theta_m_obs) -> theta_m_obs/1, Desacoplamiento de torque de gravedad/2(theta_m)
  Mux/1 -> v_abcs/1
  Subsistema físico no lineal/3(i_abcs) -> Demux/1
  Subsistema físico no lineal/6(T_l) -> T_l/1
  Subsistema físico no lineal/5(omega_m) -> omega_m_simulada/1  "omega_m"

== system consigna_5_2/5.2.5 ==
  note: CONTROLADOR
  T_per : Inport
  Tº_amb : Inport  Port=2
  q1* : Inport  Port=3
  Calculo rs : Subsystem
  Constant5 : Constant  Value=0
  Controlador PID : Subsystem
  Demux : Demux  Outputs=3
  Desacoplamiento de torque de gravedad : Subsystem
  Desacoplamientos físicos : Subsystem
  Gain5 : Gain  Gain=P_p
  Inversión de tensión : Subsystem
  Modulador de corriente : Subsystem
  Modulador de torque : Subsystem
  Mux : Mux  Inputs=3
  Mux1 : Mux  Inputs=2
  Observador de estado mejorado : Subsystem
  Sensores : Subsystem
  Setpoint : Subsystem
  Subsistema físico no lineal : Subsystem
      settings: PortSchema="{\"entries\":[{\"content\":{\"sides\":[{\"content\":{\"connectorIds\":[\"In1\",\"In2\",\"In3\",\"In4\",\"In5\"]},\"type\":\"ConnectorPlacement.EquallySpacedRectSide\",\"uuid\":\"67117692-d9ee-40bf-88b2-d8f6a60dc3b5\"},{\"content\":{\"connectorIds\":[\"Out1\",\"Out2\",\"Out3\"],\"side\":\"RIGHT\"},\"type\":\"ConnectorPlacement.EquallySpacedRectSide\",\"uuid\":\"ca2dbe86-e86f-47c7-8eac-1e82e6a5dbc0\"},{\"content\":{\"connectorIds\":[\"Out4\",\"Out5\",\"Out6\"],\"side\":\"TOP\"},\"type\":\"ConnectorPlacement.EquallySpacedRectSide\",\"uuid\":\"fbd4a5c3-5162-48dd-8002-932f8e6631f6\"}]},\"type\":\"ConnectorPlacement.EquallySpacedConnector\",\"uuid\":\"e55c07f0-88b9-4508-920f-2bf50421126b\"}],\"packageUris\":[\"http://schema.mathworks.com/mf0/Connector/R2020b\"],\"version\":\"1.0\"}"
  TD_PARK : MATLAB Function  TreatAsAtomicUnit=on
  TI_PARK1 : MATLAB Function  TreatAsAtomicUnit=on
  T_l : Outport
  T_m : Outport  Port=2
  "theta_m " : Outport  Port=3
  T_s : Outport  Port=4
  fas : Outport  Port=5
  fbs : Outport  Port=6
  fcs : Outport  Port=7
  v_abcs : Outport  Port=8
  omega_m : Outport  Port=9
  omega_theta_m_obs : Outport  Port=10
  wires:
  Inversión de tensión/1(v_as) -> Subsistema físico no lineal/2(v_as), Mux/1
  TD_PARK/3(f0s) -> Modulador de corriente/6(i_0s), Desacoplamientos físicos/6(i_0s)  "i_0s"
  TI_PARK1/1(fas) -> Inversión de tensión/1(v_as*)
  Inversión de tensión/2(v_bs) -> Subsistema físico no lineal/3(v_bs), Mux/2
  TD_PARK/1(fqs) -> Modulador de corriente/4(i_qs), Desacoplamientos físicos/4(i_qs)  "i_qs^r"
  Gain5/1 -> TD_PARK/4(theta_r), TI_PARK1/4(theta_r)
  TI_PARK1/2(fbs) -> Inversión de tensión/2(v_bs*)
  TD_PARK/2(fds) -> Modulador de torque/2(ids), Modulador de corriente/5(i_ds), Desacoplamientos físicos/5(i_ds)  "i_ds^r"
  Desacoplamientos físicos/3(v_0s*') -> TI_PARK1/3(f0s)
  Inversión de tensión/3(v_cs) -> Subsistema físico no lineal/4(v_cs), Mux/3
  Subsistema físico no lineal/1(theta_m) -> Sensores/1(theta_m)
  Subsistema físico no lineal/2(T_s) -> Sensores/2(T_s)
  Sensores/5(i_cs_medida) -> fcs/1, TD_PARK/3(fcs)
  Demux/1 -> Sensores/3(i_as)
  Modulador de torque/1(iq*) -> Modulador de corriente/1(I_qs*)
  Sensores/4(i_bs_medida) -> fbs/1, TD_PARK/2(fbs)
  Subsistema físico no lineal/5(T_m) -> T_m/1
  Modulador de corriente/1(v_qs*) -> Desacoplamientos físicos/1(v_qs*)
  Constant5/1 -> Modulador de corriente/3(I_0s*), Modulador de corriente/2(I_ds*)
  T_per/1 -> Subsistema físico no lineal/1(T_per)
  Demux/2 -> Sensores/4(i_bs)
  Modulador de corriente/3(v_0s*) -> Desacoplamientos físicos/3(v_0s*)
  Demux/3 -> Sensores/5(i_cs)
  Sensores/1(theta_m_medida) -> "theta_m "/1, Observador de estado mejorado/2(theta_m), Gain5/1
  Desacoplamientos físicos/1(v_qs*') -> TI_PARK1/1(fqs)
  Sensores/3(i_as_medida) -> TD_PARK/1(fas), fas/1
  TI_PARK1/3(fcs) -> Inversión de tensión/3(v_cs*)
  Desacoplamientos físicos/2(v_ds*') -> TI_PARK1/2(fds)
  Modulador de corriente/2(v_ds*) -> Desacoplamientos físicos/2(v_ds*)
  Setpoint/2(omega_m*) -> Controlador PID/1(omega_m*)
  q1*/1 -> Setpoint/1(q1*)
  Controlador PID/1(Tm*) -> Observador de estado mejorado/1(T_m*), Desacoplamiento de torque de gravedad/1(Tm*)
  Observador de estado mejorado/1(omega_m_obs) -> Mux1/1, Modulador de torque/3(omega_m), Controlador PID/2(omega_m), Desacoplamientos físicos/7(omega_m)
  Tº_amb/1 -> Subsistema físico no lineal/5(Tº_amb)
  Sensores/2(T_s_medida) -> Calculo rs/1(Ts), T_s/1
  Calculo rs/1(r_s) -> Desacoplamientos físicos/8(r_s)
  Desacoplamiento de torque de gravedad/1(Tm*') -> Modulador de torque/1(Tm*)
  Observador de estado mejorado/2(theta_m_obs) -> Mux1/2, Desacoplamiento de torque de gravedad/2(theta_m)
  Mux/1 -> v_abcs/1
  Subsistema físico no lineal/4(omega_m) -> omega_m/1  "omega_m"
  Subsistema físico no lineal/3(i_abcs) -> Demux/1
  Subsistema físico no lineal/6(T_l) -> T_l/1
  Mux1/1 -> omega_theta_m_obs/1

== system consigna_5_2/5.2.5' ==
  note: CONTROLADOR
  T_per : Inport
  Tº_amb : Inport  Port=2
  q1* : Inport  Port=3
  Calculo rs : Subsystem
  Constant5 : Constant  Value=0
  Controlador PID : Subsystem
  Demux : Demux  Outputs=3
  Desacoplamiento de torque de gravedad : Subsystem
  Desacoplamientos físicos : Subsystem
  Gain5 : Gain  Gain=P_p
  Inversión de tensión : Subsystem
  Modulador de corriente : Subsystem
  Modulador de torque : Subsystem
  Mux1 : Mux  Inputs=2
  Observador de estado reducido : Subsystem
  Sensores : Subsystem
  Setpoint : Subsystem
  Subsistema físico no lineal : Subsystem
      settings: PortSchema="{\"entries\":[{\"content\":{\"sides\":[{\"content\":{\"connectorIds\":[\"In1\",\"In2\",\"In3\",\"In4\",\"In5\"]},\"type\":\"ConnectorPlacement.EquallySpacedRectSide\",\"uuid\":\"67117692-d9ee-40bf-88b2-d8f6a60dc3b5\"},{\"content\":{\"connectorIds\":[\"Out1\",\"Out2\",\"Out3\"],\"side\":\"RIGHT\"},\"type\":\"ConnectorPlacement.EquallySpacedRectSide\",\"uuid\":\"ca2dbe86-e86f-47c7-8eac-1e82e6a5dbc0\"},{\"content\":{\"connectorIds\":[\"Out4\",\"Out5\",\"Out6\"],\"side\":\"TOP\"},\"type\":\"ConnectorPlacement.EquallySpacedRectSide\",\"uuid\":\"fbd4a5c3-5162-48dd-8002-932f8e6631f6\"}]},\"type\":\"ConnectorPlacement.EquallySpacedConnector\",\"uuid\":\"e55c07f0-88b9-4508-920f-2bf50421126b\"}],\"packageUris\":[\"http://schema.mathworks.com/mf0/Connector/R2020b\"],\"version\":\"1.0\"}"
  TD_PARK : MATLAB Function  TreatAsAtomicUnit=on
  TI_PARK1 : MATLAB Function  TreatAsAtomicUnit=on
  T_l : Outport
  T_m : Outport  Port=2
  "theta_m " : Outport  Port=3
  T_s : Outport  Port=4
  fas : Outport  Port=5
  fbs : Outport  Port=6
  fcs : Outport  Port=7
  v_as : Outport  Port=8
  omega_theta_obs : Outport  Port=9
  omega_m : Outport  Port=10
  v_bs : Outport  Port=11
  v_cs : Outport  Port=12
  wires:
  TD_PARK/3(f0s) -> Modulador de corriente/6(i_0s), Desacoplamientos físicos/6(i_0s)  "i_0s"
  TI_PARK1/1(fas) -> Inversión de tensión/1(v_as*)
  Inversión de tensión/2(v_bs) -> v_bs/1, Subsistema físico no lineal/3(v_bs)
  TD_PARK/1(fqs) -> Modulador de corriente/4(i_qs), Desacoplamientos físicos/4(i_qs)  "i_qs^r"
  Gain5/1 -> TD_PARK/4(theta_r), TI_PARK1/4(theta_r)
  TI_PARK1/2(fbs) -> Inversión de tensión/2(v_bs*)
  TD_PARK/2(fds) -> Modulador de torque/2(ids), Modulador de corriente/5(i_ds), Desacoplamientos físicos/5(i_ds)  "i_ds^r"
  Desacoplamientos físicos/3(v_0s*') -> TI_PARK1/3(f0s)
  Inversión de tensión/3(v_cs) -> v_cs/1, Subsistema físico no lineal/4(v_cs)
  Subsistema físico no lineal/1(theta_m) -> Sensores/1(theta_m)
  Subsistema físico no lineal/2(T_s) -> Sensores/2(T_s)
  Sensores/5(i_cs_medida) -> fcs/1, TD_PARK/3(fcs)
  Demux/1 -> Sensores/3(i_as)
  Modulador de torque/1(iq*) -> Modulador de corriente/1(I_qs*)
  Sensores/4(i_bs_medida) -> fbs/1, TD_PARK/2(fbs)
  Subsistema físico no lineal/5(T_m) -> T_m/1
  Modulador de corriente/1(v_qs*) -> Desacoplamientos físicos/1(v_qs*)
  Constant5/1 -> Modulador de corriente/3(I_0s*), Modulador de corriente/2(I_ds*)
  T_per/1 -> Subsistema físico no lineal/1(T_per)
  Demux/2 -> Sensores/4(i_bs)
  Modulador de corriente/3(v_0s*) -> Desacoplamientos físicos/3(v_0s*)
  Demux/3 -> Sensores/5(i_cs)
  Sensores/1(theta_m_medida) -> "theta_m "/1, Observador de estado reducido/2(theta_m), Gain5/1
  Desacoplamientos físicos/1(v_qs*') -> TI_PARK1/1(fqs)
  Sensores/3(i_as_medida) -> TD_PARK/1(fas), fas/1
  TI_PARK1/3(fcs) -> Inversión de tensión/3(v_cs*)
  Desacoplamientos físicos/2(v_ds*') -> TI_PARK1/2(fds)
  Modulador de corriente/2(v_ds*) -> Desacoplamientos físicos/2(v_ds*)
  Setpoint/2(omega_m*) -> Controlador PID/1(omega_m*)
  q1*/1 -> Setpoint/1(q1*)
  Controlador PID/1(Tm*) -> Observador de estado reducido/1(T_m*), Desacoplamiento de torque de gravedad/1(Tm*)
  Observador de estado reducido/1(omega_m_obs) -> Mux1/1, Modulador de torque/3(omega_m), Controlador PID/2(omega_m), Desacoplamientos físicos/7(omega_m)
  Tº_amb/1 -> Subsistema físico no lineal/5(Tº_amb)
  Sensores/2(T_s_medida) -> Calculo rs/1(Ts), T_s/1
  Calculo rs/1(r_s) -> Desacoplamientos físicos/8(r_s)
  Desacoplamiento de torque de gravedad/1(Tm*') -> Modulador de torque/1(Tm*)
  Observador de estado reducido/2(theta_m_obs) -> Mux1/2, Desacoplamiento de torque de gravedad/2(theta_m)
  Inversión de tensión/1(v_as) -> Subsistema físico no lineal/2(v_as), v_as/1
  Mux1/1 -> omega_theta_obs/1
  Subsistema físico no lineal/4(omega_m) -> omega_m/1  "omega_m"
  Subsistema físico no lineal/6(T_l) -> T_l/1
  Subsistema físico no lineal/3(i_abcs) -> Demux/1
